simulink model "SystemModel"  (R2026a)
settings: Solver=FixedStepDiscrete  StopTime=inf  FixedStep=ts_system  EnableMultiTasking=on
StartFcn:
  | Simulink.sdi.setRecordData(false);
undefined symbols (not defined in the file): Battery, BCE12, BCE_Set_init, BMS_Controller_State, Cell10_P, Cell11_P, Cell12_P, Cell1_N, Cell1_P, Cell2_P, Cell3_P, Cell4_P, Cell5_P, Cell6_P, Cell7_P, Cell8_P, Cell9_P, Cell_Temperatures, Cell_Voltages, Charging_State, currentFactor, CV_Gain, Device_01, DiscIntNeverNeededParam, I_cc, MaxCellVoltThrsld, noCurrent, Ns_Module, NumModules, OverCellVoltageLimit, sg_bce, SOCInit, SRE, ts_controller, ts_system, UnderCellVoltageLimit, voltThreshold
libraries: slrealtimeethercatlib x99, fl_lib x65, nesl_utility x43, simulink x23, slrealtimeutilitieslib x13, sl_discontinuities x13, dspstat3 x12, canmsglib x11, speedgoatlib_IO611 x9, batt_lib x3, sharedTrackingLibrary x2, BatteryModuleLibrary_12Cells_lib x1
(part 1 of 6)
settings Model: DataDictionary=System.sldd  ExtModeEnableFloating=off  Creator=The MathWorks, Inc.  LastModifiedBy=jatin.anand
settings SolverCC: ConcurrentTasks=on  PositivePriorityOrder=on  InsertRTBMode=Never (minimum delay)
settings DataIOCC: ExternalInput=off  InitialState=off  SignalLoggingName=logsOut
settings OptimizationCC: BooleanDataType=off  DefaultUnderspecifiedDataType=single  OptimizeBlockIOStorage=off  PassReuseOutputArgsThreshold=0.0  InitFltsAndDblsToZero=on
settings DebuggingCC: SignalInfNanChecking=error  SaveWithParameterizedLinksMsg=none  CheckExecutionContextPreStartOutputMsg=on  SignalResolutionControl=TryResolveAllWithWarning  InheritedTsInSrcMsg=none  TasksWithSamePriorityMsg=none  IntegerOverflowMsg=error  ParameterPrecisionLossMsg=none
settings HardwareCC: ProdBitPerLong=64.0  ProdHWDeviceType=Intel->x86-64 (Linux 64)
settings ModelReferenceCC: ModelReferenceNumInstancesAllowed=Single
settings RTWCC: SystemTargetFile=speedgoat.tlc  TemplateMakefile=slrealtime_default_tmf  GenerateReport=on  Toolchain=Simulink Real-Time Toolchain  BuildConfiguration=Faster Runs  TargetLang=C++  Description=Speedgoat Real-Time Target Machine
settings CodeAppCC: MaxIdLength=51.0
settings SimulinkRealTimeTargetCC: SLRTFileLogMaxRuns=1.0  MultiwordLength=2048.0
settings SimscapeCC: SimscapeNominalValues="[{\"value\":\"1\",\"unit\":\"A\"},{\"value\":\"1\",\"unit\":\"bar\"},{\"value\":\"1\",\"unit\":\"cm^2\"},{\"value\":\"1\",\"unit\":\"cm^3/s\"},{\"value\":\"1\",\"unit\":\"kJ/kg\"},{\"value\":\"1\",\"unit\":\"kW\"},{\"value\":\"1\",\"unit\":\"l\"},{\"value\":\"1\",\"unit\":\"N\"},{\"value\":\"1\",\"unit\":\"N*m\"},{\"value\":\"1\",\"unit\":\"V\"}]"  SimscapeLogType=none  SimscapeLogDataHistory=5000.0

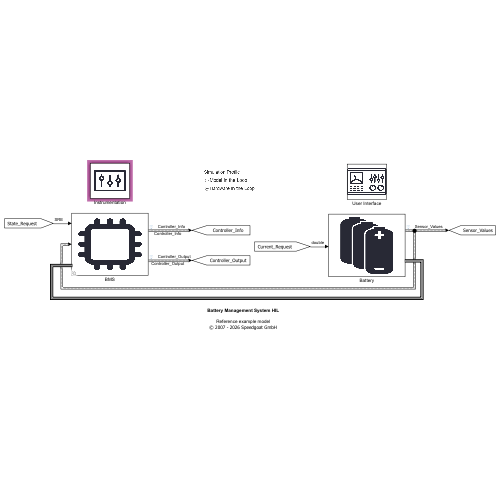
[thumbnail: Simulink's stored preview of the top-level diagram]
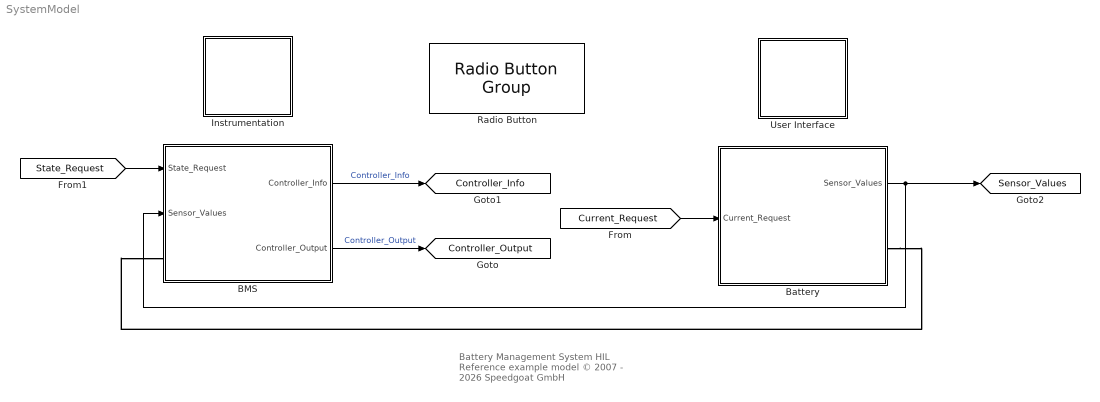
== system SystemModel ==
  note: Battery Management System HIL
      |
      | Reference example model
      | © 2007 - 2026 Speedgoat GmbH
  BMS : Subsystem  Variant=on  VariantControl=Choice
      mask Display: image('BMS.png'); % Use "Edit Image" on toolstrip to change.
  Battery : Subsystem
      mask Display: image('battery.png'); % Use "Edit Image" on toolstrip to change.
  Instrumentation : Subsystem
      mask Display: image('tunable.png'); % Use "Edit Image" on toolstrip to change.
  Radio Button : RadioButtonGroup  LabelPosition=Hide  SelectedLabel=Hardware-in-the-Loop  ButtonGroupName=Simulation Profile
  User Interface : Subsystem
      mask Display: image('UI.png'); % Use "Edit Image" on toolstrip to change.
  tag scope: Controller_Info=global, Controller_Output=global, Sensor_Values=global
  wires:
  [Current_Request] -> Battery/1(Current_Request)
  Battery/1(Sensor_Values) -> [Sensor_Values], BMS/2(Sensor_Values)
  BMS/1(Controller_Info) -> [Controller_Info]  "Controller_Info"
  BMS/2(Controller_Output) -> [Controller_Output]  "Controller_Output"
  [State_Request] -> BMS/1(State_Request)
  connections:
  Battery/RConn1 -- BMS/LConn1

== system SystemModel/BMS ==
  State_Request : Inport
  Sensor_Values : Inport  Port=2
  HIL : Subsystem  VariantControl=strcmp(get_param([bdroot '/Instrumentation/Simulation_Profile_Value'], 'Value'),'1')
  MIL : Subsystem  VariantControl=strcmp(get_param([bdroot '/Instrumentation/Simulation_Profile_Value'], 'Value'),'0')
  Cells : PMIOPort  Side=Left
  Controller_Info : Outport
  Controller_Output : Outport  Port=2

== system SystemModel/Battery ==
  Current_Request : Inport
  Battery Pack : Subsystem
  Bus Creator : BusCreator  Inputs=4  OutDataTypeStr=Bus: Sensor_Values  NonVirtualBus=on
      settings: InheritFromInputs=off
  Bypass : Subsystem
  Data Type Conversion{,1..3} (4 alike) : DataTypeConversion  OutDataTypeStr=single  SaturateOnIntegerOverflow=off  RndMeth=Floor
  Electrical Interface : Subsystem
  HW Interface : Subsystem  Variant=on  VariantControl=Choice
  Rate Transition1 : RateTransition  OutPortSampleTime=ts_system
  Cells : PMIOPort  Side=Right
  Sensor_Values : Outport
  tag scope: Cells_SOCs=global
  wires:
  Current_Request/1 -> Rate Transition1/1
  Electrical Interface/1(Pack_Current) -> Data Type Conversion2/1
  Electrical Interface/2(Pack_Voltage) -> Data Type Conversion1/1
  Data Type Conversion/1 -> Bus Creator/1  "Cell_Voltages"
  Data Type Conversion1/1 -> Bus Creator/4  "Pack_Voltage"
  Data Type Conversion2/1 -> Bus Creator/3  "Pack_Current"
  Data Type Conversion3/1 -> Bus Creator/2  "Cell_Temperatures"
  [Ambient_Temperature_User] -> Battery Pack/1(Ambient_Temperature)
  Battery Pack/1(Cell_Voltages) -> Data Type Conversion/1
  Battery Pack/2(Cell_Temperatures) -> Data Type Conversion3/1
  Battery Pack/3(Cell_SOCs) -> [Cells_SOCs]  "Cell_SOCs"
  Bus Creator/1 -> Bypass/1(IN)
  HW Interface/1(Sensor_Values_Real) -> Sensor_Values/1
  Rate Transition1/1 -> Electrical Interface/1(Current_Request)
  Bypass/1(OUT) -> HW Interface/1(Sensor_Values_Sim)
  [Short_Circuits_User] -> Battery Pack/2(Short_Circuits)
  connections:
  Battery Pack/RConn1 -- Electrical Interface/LConn1
  Battery Pack/RConn2 -- Electrical Interface/LConn2
  Battery Pack/RConn3 -- HW Interface/LConn1
  HW Interface/RConn1 -- Cells/RConn1

== system SystemModel/Instrumentation ==
  Ambient_Temperature : Constant  Value=25
  Celsius_to_Kelvin : Subsystem
  Constant1 : Constant
  Current : Constant  Value=-20
  Current Control : Subsystem
  Instrumented Signals : Subsystem
  Simulation_Profile_Value : Constant
  State_Request : simulink/Sources/Enumerated Constant  OutDataTypeStr=Enum: SRE  Value=SRE.Standby  SampleTime=inf
  Terminator4 : Terminator
  tag scope: Ambient_Temperature_User=global, Broken_Wires_User=global, Current_Request=global, Short_Circuits_User=global, State_Request=global
  wires:
  Celsius_to_Kelvin/1(K) -> [Ambient_Temperature_User]
  Ambient_Temperature/1 -> Celsius_to_Kelvin/1(C)
  Current/1 -> Current Control/1(Current_Request_User)
  Constant1/1 -> Current Control/2(Current_Request_User_Bypass)
  Current Control/1(Current_Request) -> [Current_Request]  "Pack_Current_Request"
  State_Request/1 -> [State_Request]
  [Controller_Output] -> Instrumented Signals/1(Controller_Output), Current Control/4(Controller_Output)
  [Controller_Info] -> Instrumented Signals/2(Controller_Info), Current Control/3(Controller_Info)
  [Sensor_Values] -> Instrumented Signals/3(Sensor_Values)
  [Balancing_Currents] -> Instrumented Signals/4(Balancing_Currents)
  [Cells_SOCs] -> Instrumented Signals/5(Cells_SOCs)
  Instrumented Signals/1(Short-Circuits) -> [Short_Circuits_User]
  Instrumented Signals/2(Broken_Wires) -> [Broken_Wires_User]
  Simulation_Profile_Value/1 -> Terminator4/1
